simulink model "PassengerCar"  (R2019b)
settings: Solver=ode1  StartTime=0  StopTime=25  FixedStep=1.0000000000000000e-003  RelTol=1e-3
InitFcn:
  | sampleTime = str2double(get_param(bdroot, 'FixedStep'));
undefined symbols (not defined in the file or in its folder): AccPedalPos, BrakePedalPos, BrakeSwitch, DiscIntNeverNeededParam, DYNA4, EngSpd, IgnitionSwitch, InitialGear, InitialSpeed, IntendedEngTrq, LeftIndicator, MainBrakePress, MaxGear, MDL, MinGear, RefAcc, RefLane, RefLatPos, RefPath, RefPathCurv, RefSpd, RefSpdPreview, RefSpdRetrospect, RightIndicator, SteeringWheelAng, SteeringWheelTrq, UserDefinedRefValue, vm_const
libraries: UtilitiesLibrary x31, simulink x18, WheelSystemModules x13, LongitudinalControllerModules x13, LateralControllerModules x7, AnimationBusselectorModules x5, EnvironmentModules x5, BasicEngineControlModules x5, MiscellaneousControlModules x5, Animation3Modules x4, AuxiliariesModules x4, TireModules x4
(part 16 of 39)

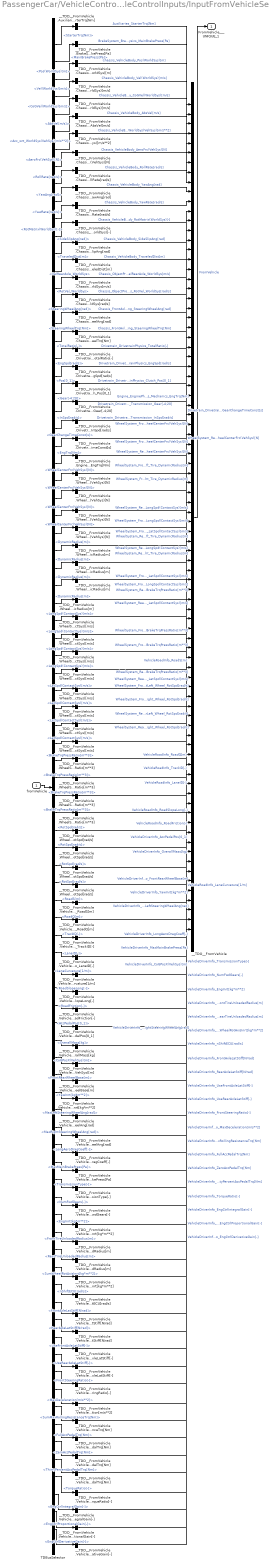
== system PassengerCar/VehicleControl/VehicleControlInputs/InputFromVehicleSelection ==
  fromVehicle : Inport
  TDBusSelector : BusSelector  OutputSignals=Auxiliaries.StarterTrq[Nm],BrakeSystem.BrakeSystemPhysics.MainBrakePress[Pa],Chassis.VehicleBody.Pos(WorldSys)[m],Chassis.VehicleBody.Vel(WorldSys)[m/s],Chassis.VehicleBody.CoGVel(WorldSys)[m/s],Chassis.VehicleBody.AbsVel[m/s],Chassis.VehicleBody.Acc_wrt_WorldSys(VehSys)[m/s**2],Chassis.VehicleBody.AeroFrc(VehSys)[N],Chassis.VehicleBody.RollRate[rad/s],Chassis.VehicleBody.YawAng[rad],Chassis.VehicleBody.YawRate[rad/s],Chassis.VehicleBody.RotMatrix(WorldSys)[-],Chassis.VehicleBody.SideSlipAng[rad],Chassis.VehicleBody.TraveledDist[m],Chassis.ObjectProperties.VelRearAxle_WorldSys,Chassis.ObjectProperties.RotVel_WorldSys,Chassis.FrontAxle.Steering.SteeringWheelAng[rad],Chassis.FrontAxle.Steering.SteeringWheelTrq[Nm],Drivetrain.DrivetrainPhysics.TotalRatio[-],Drivetrain.DrivetrainPhysics.EngSpd[rad/s],Drivetrain.DrivetrainPhysics.Clutch.Pos[0_1],Drivetrain.DrivetrainPhysics.Transmission.Gear[-4;20],Drivetrain.DrivetrainPhysics.Transmission.InSpd[rad/s],Drivetrain.DrivetrainPhysics.Transmission.GearChangeTimeConst[s],Engine.EnginePhysics.Mechanics.EngTrq[Nm],WheelSystem.FrontLeft.Tire.WheelCenterFrc(VehSys)[N],WheelSystem.FrontRight.Tire.WheelCenterFrc(VehSys)[N],WheelSystem.RearLeft.Tire.WheelCenterFrc(VehSys)[N],WheelSystem.RearRight.Tire.WheelCenterFrc(VehSys)[N],WheelSystem.FrontLeft.Tire.DynamicRadius[m],WheelSystem.FrontRight.Tire.DynamicRadius[m],WheelSystem.RearLeft.Tire.DynamicRadius[m],WheelSystem.RearRight.Tire.DynamicRadius[m],WheelSystem.FrontLeft.Tire.LongSpd(ContactSys)[m/s],WheelSystem.FrontRight.Tire.LongSpd(ContactSys)[m/s],WheelSystem.RearLeft.Tire.LongSpd(ContactSys)[m/s],WheelSystem.RearRight.Tire.LongSpd(ContactSys)[m/s],WheelSystem.FrontLeft.Tire.LatSpd(ContactSys)[m/s],WheelSystem.FrontRight.Tire.LatSpd(ContactSys)[m/s],WheelSystem.RearLeft.Tire.LatSpd(ContactSys)[m/s],WheelSystem.RearRight.Tire.LatSpd(ContactSys)[m/s],WheelSystem.FrontLeft.Wheel.BrakeTrqPressRatio[m**3],WheelSystem.FrontRight.Wheel.BrakeTrqPressRatio[m**3],WheelSystem.RearLeft.Wheel.BrakeTrqPressRatio[m**3],WheelSystem.RearRight.Wheel.BrakeTrqPressRatio[m**3],WheelSystem.FrontLeft.Wheel.RotSpd[rad/s],WheelSystem.FrontRight.Wheel.RotSpd[rad/s],WheelSystem.RearLeft.Wheel.RotSpd[rad/s],WheelSystem.RearRight.Wheel.RotSpd[rad/s],VehicleRoadInfo.RoadS[m],VehicleRoadInfo.RoadQ[m],VehicleRoadInfo.TrackID[-],VehicleRoadInfo.LaneID[-],VehicleRoadInfo.LaneCurvature[1/m],VehicleRoadInfo.RoadSlopeLong[-],VehicleRoadInfo.RoadFriction[-],VehicleDriverInfo.AccPedalPos[0_1],VehicleDriverInfo.OverallMass[kg],VehicleDriverInfo.CoGPosX(VehSys)[m],VehicleDriverInfo.FrontRearWheelBase[m],VehicleDriverInfo.YawInrt[kg*m**2],VehicleDriverInfo.MaxLeftSteeringWheelAng[rad],VehicleDriverInfo.MaxRightSteeringWheelAng[rad],VehicleDriverInfo.LongAeroDragCoeff[-],VehicleDriverInfo.MaxMainBrakePress[Pa],VehicleDriverInfo.TransmissionType[-],VehicleDriverInfo.NumFwdGears[-],VehicleDriverInfo.EngInrt[kg*m**2],VehicleDriverInfo.FrontTireUnloadedRadius[m],VehicleDriverInfo.RearTireUnloadedRadius[m],VehicleDriverInfo.SumWheelRotAxisInrt[kg*m**2],VehicleDriverInfo.nShiftECU[rad/s],VehicleDriverInfo.FrontAxleLatStiff[N/rad],VehicleDriverInfo.RearAxleLatStiff[N/rad],VehicleDriverInfo.UseFrontAxleLatStiff[-],VehicleDriverInfo.UseRearAxleLatStiff[-],VehicleDriverInfo.FrontSteeringRatio[-],VehicleDriverInfo.MaxDeceleration[m/s**2],VehicleDriverInfo.SumMaxRollingResistanceTrq[Nm],VehicleDriverInfo.FullAccPedalTrq[Nm],VehicleDriverInfo.ZeroAccPedalTrq[Nm],VehicleDriverInfo.ThirtyPercentAccPedalTrq[Nm],VehicleDriverInfo.TorqueRatio[-],VehicleDriverInfo.EngCtrlIntegralGain[-],VehicleDriverInfo.EngCtrlProportionalGain[-],VehicleDriverInfo.EngCtrlDerivativeGain[-]
  __TDD__FromVehicle.Auxiliaries_StarterTrq[Nm] : Demux  Outputs=[1]
  __TDD__FromVehicle.BrakeSystem_BrakeSystemPhysics_MainBrakePress[Pa] : Demux  Outputs=[1]
  __TDD__FromVehicle.Chassis_FrontAxle_Steering_SteeringWheelAng[rad] : Demux  Outputs=[1]
  __TDD__FromVehicle.Chassis_FrontAxle_Steering_SteeringWheelTrq[Nm] : Demux  Outputs=1
  __TDD__FromVehicle.Chassis_ObjectProperties_RotVel_WorldSys[rad/s] : Demux  Outputs=[3]
  __TDD__FromVehicle.Chassis_ObjectProperties_VelRearAxle_WorldSys[m/s] : Demux  Outputs=[3]
  __TDD__FromVehicle.Chassis_VehicleBody_AbsVel[m/s] : Demux  Outputs=[1]
  __TDD__FromVehicle.Chassis_VehicleBody_Acc_wrt_WorldSys(VehSys)[m/s**2] : Demux  Outputs=[3]
  __TDD__FromVehicle.Chassis_VehicleBody_AeroFrc(VehSys)[N] : Demux  Outputs=[3]
  __TDD__FromVehicle.Chassis_VehicleBody_CoGVel(WorldSys)[m/s] : Demux  Outputs=[3]
  __TDD__FromVehicle.Chassis_VehicleBody_Pos(WorldSys)[m] : Demux  Outputs=[3]
  __TDD__FromVehicle.Chassis_VehicleBody_RollRate[rad/s] : Demux  Outputs=[1]
  __TDD__FromVehicle.Chassis_VehicleBody_RotMatrix(WorldSys)[-] : Demux  Outputs=[9]
  __TDD__FromVehicle.Chassis_VehicleBody_SideSlipAng[rad] : Demux  Outputs=[1]
  __TDD__FromVehicle.Chassis_VehicleBody_TraveledDist[m] : Demux  Outputs=[1]
  __TDD__FromVehicle.Chassis_VehicleBody_Vel(WorldSys)[m/s] : Demux  Outputs=[3]
  __TDD__FromVehicle.Chassis_VehicleBody_YawAng[rad] : Demux  Outputs=[1]
  __TDD__FromVehicle.Chassis_VehicleBody_YawRate[rad/s] : Demux  Outputs=[1]
  __TDD__FromVehicle.Drivetrain_DrivetrainPhysics_Clutch_Pos[0_1] : Demux  Outputs=[1]
  __TDD__FromVehicle.Drivetrain_DrivetrainPhysics_EngSpd[rad/s] : Demux  Outputs=[1]
  __TDD__FromVehicle.Drivetrain_DrivetrainPhysics_TotalRatio[-] : Demux  Outputs=[1]
  __TDD__FromVehicle.Drivetrain_DrivetrainPhysics_Transmission_GearChangeTimeConst[s] : Demux  Outputs=[1]
  __TDD__FromVehicle.Drivetrain_DrivetrainPhysics_Transmission_Gear[-4;20] : Demux  Outputs=[1]
  __TDD__FromVehicle.Drivetrain_DrivetrainPhysics_Transmission_InSpd[rad/s] : Demux  Outputs=[1]
  __TDD__FromVehicle.Engine_EnginePhysics_Mechanics_EngTrq[Nm] : Demux  Outputs=[1]
  __TDD__FromVehicle.VehicleDriverInfo_AccPedalPos[0_1] : Demux  Outputs=[1]
  __TDD__FromVehicle.VehicleDriverInfo_CoGPosX(VehSys)[m] : Demux  Outputs=[1]
  __TDD__FromVehicle.VehicleDriverInfo_EngCtrlDerivativeGain[-] : Demux  Outputs=[1]
  __TDD__FromVehicle.VehicleDriverInfo_EngCtrlIntegralGain[-] : Demux  Outputs=[1]
  __TDD__FromVehicle.VehicleDriverInfo_EngCtrlProportionalGain[-] : Demux  Outputs=[1]
  __TDD__FromVehicle.VehicleDriverInfo_EngInrt[kg*m**2] : Demux  Outputs=[1]
  __TDD__FromVehicle.VehicleDriverInfo_FrontAxleLatStiff[N/rad] : Demux  Outputs=[1]
  __TDD__FromVehicle.VehicleDriverInfo_FrontRearWheelBase[m] : Demux  Outputs=[1]
  __TDD__FromVehicle.VehicleDriverInfo_FrontSteeringRatio[-] : Demux  Outputs=[1]
  __TDD__FromVehicle.VehicleDriverInfo_FrontTireUnloadedRadius[m] : Demux  Outputs=[1]
  __TDD__FromVehicle.VehicleDriverInfo_FullAccPedalTrq[Nm] : Demux  Outputs=[1]
  __TDD__FromVehicle.VehicleDriverInfo_LongAeroDragCoeff[-] : Demux  Outputs=[1]
  __TDD__FromVehicle.VehicleDriverInfo_MaxDeceleration[m/s**2] : Demux  Outputs=[1]
  __TDD__FromVehicle.VehicleDriverInfo_MaxLeftSteeringWheelAng[rad] : Demux  Outputs=[1]
  __TDD__FromVehicle.VehicleDriverInfo_MaxMainBrakePress[Pa] : Demux  Outputs=[1]
  __TDD__FromVehicle.VehicleDriverInfo_MaxRightSteeringWheelAng[rad] : Demux  Outputs=[1]
  __TDD__FromVehicle.VehicleDriverInfo_NumFwdGears[-] : Demux  Outputs=[1]
  __TDD__FromVehicle.VehicleDriverInfo_OverallMass[kg] : Demux  Outputs=[1]
  __TDD__FromVehicle.VehicleDriverInfo_RearAxleLatStiff[N/rad] : Demux  Outputs=[1]
  __TDD__FromVehicle.VehicleDriverInfo_RearTireUnloadedRadius[m] : Demux  Outputs=[1]
  __TDD__FromVehicle.VehicleDriverInfo_SumMaxRollingResistanceTrq[Nm] : Demux  Outputs=[1]
  __TDD__FromVehicle.VehicleDriverInfo_SumWheelRotAxisInrt[kg*m**2] : Demux  Outputs=[1]
  __TDD__FromVehicle.VehicleDriverInfo_ThirtyPercentAccPedalTrq[Nm] : Demux  Outputs=[1]
  __TDD__FromVehicle.VehicleDriverInfo_TorqueRatio[-] : Demux  Outputs=[1]
  __TDD__FromVehicle.VehicleDriverInfo_TransmissionType[-] : Demux  Outputs=[1]
  __TDD__FromVehicle.VehicleDriverInfo_UseFrontAxleLatStiff[-] : Demux  Outputs=[1]
  __TDD__FromVehicle.VehicleDriverInfo_UseRearAxleLatStiff[-] : Demux  Outputs=[1]
  __TDD__FromVehicle.VehicleDriverInfo_YawInrt[kg*m**2] : Demux  Outputs=[1]
  __TDD__FromVehicle.VehicleDriverInfo_ZeroAccPedalTrq[Nm] : Demux  Outputs=[1]
  __TDD__FromVehicle.VehicleDriverInfo_nShiftECU[rad/s] : Demux  Outputs=[1]
  __TDD__FromVehicle.VehicleRoadInfo_LaneCurvature[1/m] : Demux  Outputs=[1]
  __TDD__FromVehicle.VehicleRoadInfo_LaneID[-] : Demux  Outputs=[1]
  __TDD__FromVehicle.VehicleRoadInfo_RoadFriction[-] : Demux  Outputs=[1]
  __TDD__FromVehicle.VehicleRoadInfo_RoadQ[m] : Demux  Outputs=[1]
  __TDD__FromVehicle.VehicleRoadInfo_RoadS[m] : Demux  Outputs=[1]
  __TDD__FromVehicle.VehicleRoadInfo_RoadSlopeLong[-] : Demux  Outputs=[1]
  __TDD__FromVehicle.VehicleRoadInfo_TrackID[-] : Demux  Outputs=[1]
  __TDD__FromVehicle.WheelSystem_FrontLeft_Tire_DynamicRadius[m] : Demux  Outputs=[1]
  __TDD__FromVehicle.WheelSystem_FrontLeft_Tire_LatSpd(ContactSys)[m/s] : Demux  Outputs=[1]
  __TDD__FromVehicle.WheelSystem_FrontLeft_Tire_LongSpd(ContactSys)[m/s] : Demux  Outputs=[1]
  __TDD__FromVehicle.WheelSystem_FrontLeft_Tire_WheelCenterFrc(VehSys)[N] : Demux  Outputs=[3]
  __TDD__FromVehicle.WheelSystem_FrontLeft_Wheel_BrakeTrqPressRatio[m**3] : Demux  Outputs=[1]
  __TDD__FromVehicle.WheelSystem_FrontLeft_Wheel_RotSpd[rad/s] : Demux  Outputs=[1]
  __TDD__FromVehicle.WheelSystem_FrontRight_Tire_DynamicRadius[m] : Demux  Outputs=[1]
  __TDD__FromVehicle.WheelSystem_FrontRight_Tire_LatSpd(ContactSys)[m/s] : Demux  Outputs=[1]
  __TDD__FromVehicle.WheelSystem_FrontRight_Tire_LongSpd(ContactSys)[m/s] : Demux  Outputs=[1]
  __TDD__FromVehicle.WheelSystem_FrontRight_Tire_WheelCenterFrc(VehSys)[N] : Demux  Outputs=[3]
  __TDD__FromVehicle.WheelSystem_FrontRight_Wheel_BrakeTrqPressRatio[m**3] : Demux  Outputs=[1]
  __TDD__FromVehicle.WheelSystem_FrontRight_Wheel_RotSpd[rad/s] : Demux  Outputs=[1]
  __TDD__FromVehicle.WheelSystem_RearLeft_Tire_DynamicRadius[m] : Demux  Outputs=[1]
  __TDD__FromVehicle.WheelSystem_RearLeft_Tire_LatSpd(ContactSys)[m/s] : Demux  Outputs=[1]
  __TDD__FromVehicle.WheelSystem_RearLeft_Tire_LongSpd(ContactSys)[m/s] : Demux  Outputs=[1]
  __TDD__FromVehicle.WheelSystem_RearLeft_Tire_WheelCenterFrc(VehSys)[N] : Demux  Outputs=[3]
  __TDD__FromVehicle.WheelSystem_RearLeft_Wheel_BrakeTrqPressRatio[m**3] : Demux  Outputs=[1]
  __TDD__FromVehicle.WheelSystem_RearLeft_Wheel_RotSpd[rad/s] : Demux  Outputs=[1]
  __TDD__FromVehicle.WheelSystem_RearRight_Tire_DynamicRadius[m] : Demux  Outputs=[1]
  __TDD__FromVehicle.WheelSystem_RearRight_Tire_LatSpd(ContactSys)[m/s] : Demux  Outputs=[1]
  __TDD__FromVehicle.WheelSystem_RearRight_Tire_LongSpd(ContactSys)[m/s] : Demux  Outputs=[1]
  __TDD__FromVehicle.WheelSystem_RearRight_Tire_WheelCenterFrc(VehSys)[N] : Demux  Outputs=[3]
  __TDD__FromVehicle.WheelSystem_RearRight_Wheel_BrakeTrqPressRatio[m**3] : Demux  Outputs=[1]
  __TDD__FromVehicle.WheelSystem_RearRight_Wheel_RotSpd[rad/s] : Demux  Outputs=[1]
  __TDO__FromVehicle : BusCreator  Inputs=86
  FromVehicle___UNIQUE_1 : Outport  Description=|  VectorParamsAs1DForOutWhenUnconnected=off
      | <name>Auxiliaries.StarterTrq[Nm]</name>
      | <comment>Starter torque</comment>
  wires:
  __TDO__FromVehicle/1 -> FromVehicle___UNIQUE_1/1  "FromVehicle"
  __TDD__FromVehicle.VehicleDriverInfo_EngCtrlDerivativeGain[-]/1 -> __TDO__FromVehicle/86  "VehicleDriverInfo_EngCtrlDerivativeGain[-]"
  TDBusSelector/86 -> __TDD__FromVehicle.VehicleDriverInfo_EngCtrlDerivativeGain[-]/1  "<EngCtrlDerivativeGain[-]>"
  __TDD__FromVehicle.VehicleDriverInfo_EngCtrlProportionalGain[-]/1 -> __TDO__FromVehicle/85  "VehicleDriverInfo_EngCtrlProportionalGain[-]"
  TDBusSelector/85 -> __TDD__FromVehicle.VehicleDriverInfo_EngCtrlProportionalGain[-]/1  "<EngCtrlProportionalGain[-]>"
  __TDD__FromVehicle.VehicleDriverInfo_EngCtrlIntegralGain[-]/1 -> __TDO__FromVehicle/84  "VehicleDriverInfo_EngCtrlIntegralGain[-]"
  TDBusSelector/84 -> __TDD__FromVehicle.VehicleDriverInfo_EngCtrlIntegralGain[-]/1  "<EngCtrlIntegralGain[-]>"
  __TDD__FromVehicle.VehicleDriverInfo_TorqueRatio[-]/1 -> __TDO__FromVehicle/83  "VehicleDriverInfo_TorqueRatio[-]"
  TDBusSelector/83 -> __TDD__FromVehicle.VehicleDriverInfo_TorqueRatio[-]/1  "<TorqueRatio[-]>"
  __TDD__FromVehicle.VehicleDriverInfo_ThirtyPercentAccPedalTrq[Nm]/1 -> __TDO__FromVehicle/82  "VehicleDriverInfo_ThirtyPercentAccPedalTrq[Nm]"
  TDBusSelector/82 -> __TDD__FromVehicle.VehicleDriverInfo_ThirtyPercentAccPedalTrq[Nm]/1  "<ThirtyPercentAccPedalTrq[Nm]>"
  __TDD__FromVehicle.VehicleDriverInfo_ZeroAccPedalTrq[Nm]/1 -> __TDO__FromVehicle/81  "VehicleDriverInfo_ZeroAccPedalTrq[Nm]"
  TDBusSelector/81 -> __TDD__FromVehicle.VehicleDriverInfo_ZeroAccPedalTrq[Nm]/1  "<ZeroAccPedalTrq[Nm]>"
  __TDD__FromVehicle.VehicleDriverInfo_FullAccPedalTrq[Nm]/1 -> __TDO__FromVehicle/80  "VehicleDriverInfo_FullAccPedalTrq[Nm]"
  TDBusSelector/80 -> __TDD__FromVehicle.VehicleDriverInfo_FullAccPedalTrq[Nm]/1  "<FullAccPedalTrq[Nm]>"
  __TDD__FromVehicle.VehicleDriverInfo_SumMaxRollingResistanceTrq[Nm]/1 -> __TDO__FromVehicle/79  "VehicleDriverInfo_SumMaxRollingResistanceTrq[Nm]"
  TDBusSelector/79 -> __TDD__FromVehicle.VehicleDriverInfo_SumMaxRollingResistanceTrq[Nm]/1  "<SumMaxRollingResistanceTrq[Nm]>"
  __TDD__FromVehicle.VehicleDriverInfo_MaxDeceleration[m/s**2]/1 -> __TDO__FromVehicle/78  "VehicleDriverInfo_MaxDeceleration[m/s**2]"
  TDBusSelector/78 -> __TDD__FromVehicle.VehicleDriverInfo_MaxDeceleration[m/s**2]/1  "<MaxDeceleration[m/s**2]>"
  __TDD__FromVehicle.VehicleDriverInfo_FrontSteeringRatio[-]/1 -> __TDO__FromVehicle/77  "VehicleDriverInfo_FrontSteeringRatio[-]"
  TDBusSelector/77 -> __TDD__FromVehicle.VehicleDriverInfo_FrontSteeringRatio[-]/1  "<FrontSteeringRatio[-]>"
  __TDD__FromVehicle.VehicleDriverInfo_UseRearAxleLatStiff[-]/1 -> __TDO__FromVehicle/76  "VehicleDriverInfo_UseRearAxleLatStiff[-]"
  TDBusSelector/76 -> __TDD__FromVehicle.VehicleDriverInfo_UseRearAxleLatStiff[-]/1  "<UseRearAxleLatStiff[-]>"
  __TDD__FromVehicle.VehicleDriverInfo_UseFrontAxleLatStiff[-]/1 -> __TDO__FromVehicle/75  "VehicleDriverInfo_UseFrontAxleLatStiff[-]"
  TDBusSelector/75 -> __TDD__FromVehicle.VehicleDriverInfo_UseFrontAxleLatStiff[-]/1  "<UseFrontAxleLatStiff[-]>"
  __TDD__FromVehicle.VehicleDriverInfo_RearAxleLatStiff[N/rad]/1 -> __TDO__FromVehicle/74  "VehicleDriverInfo_RearAxleLatStiff[N/rad]"
  TDBusSelector/74 -> __TDD__FromVehicle.VehicleDriverInfo_RearAxleLatStiff[N/rad]/1  "<RearAxleLatStiff[N/rad]>"
  __TDD__FromVehicle.VehicleDriverInfo_FrontAxleLatStiff[N/rad]/1 -> __TDO__FromVehicle/73  "VehicleDriverInfo_FrontAxleLatStiff[N/rad]"
  TDBusSelector/73 -> __TDD__FromVehicle.VehicleDriverInfo_FrontAxleLatStiff[N/rad]/1  "<FrontAxleLatStiff[N/rad]>"
  __TDD__FromVehicle.VehicleDriverInfo_nShiftECU[rad/s]/1 -> __TDO__FromVehicle/72  "VehicleDriverInfo_nShiftECU[rad/s]"
  TDBusSelector/72 -> __TDD__FromVehicle.VehicleDriverInfo_nShiftECU[rad/s]/1  "<nShiftECU[rad/s]>"
  __TDD__FromVehicle.VehicleDriverInfo_SumWheelRotAxisInrt[kg*m**2]/1 -> __TDO__FromVehicle/71  "VehicleDriverInfo_SumWheelRotAxisInrt[kg*m**2]"
  TDBusSelector/71 -> __TDD__FromVehicle.VehicleDriverInfo_SumWheelRotAxisInrt[kg*m**2]/1  "<SumWheelRotAxisInrt[kg*m**2]>"
  __TDD__FromVehicle.VehicleDriverInfo_RearTireUnloadedRadius[m]/1 -> __TDO__FromVehicle/70  "VehicleDriverInfo_RearTireUnloadedRadius[m]"
  TDBusSelector/70 -> __TDD__FromVehicle.VehicleDriverInfo_RearTireUnloadedRadius[m]/1  "<RearTireUnloadedRadius[m]>"
  __TDD__FromVehicle.VehicleDriverInfo_FrontTireUnloadedRadius[m]/1 -> __TDO__FromVehicle/69  "VehicleDriverInfo_FrontTireUnloadedRadius[m]"
  TDBusSelector/69 -> __TDD__FromVehicle.VehicleDriverInfo_FrontTireUnloadedRadius[m]/1  "<FrontTireUnloadedRadius[m]>"
  __TDD__FromVehicle.VehicleDriverInfo_EngInrt[kg*m**2]/1 -> __TDO__FromVehicle/68  "VehicleDriverInfo_EngInrt[kg*m**2]"
  TDBusSelector/68 -> __TDD__FromVehicle.VehicleDriverInfo_EngInrt[kg*m**2]/1  "<EngInrt[kg*m**2]>"
  __TDD__FromVehicle.VehicleDriverInfo_NumFwdGears[-]/1 -> __TDO__FromVehicle/67  "VehicleDriverInfo_NumFwdGears[-]"
  TDBusSelector/67 -> __TDD__FromVehicle.VehicleDriverInfo_NumFwdGears[-]/1  "<NumFwdGears[-]>"
  __TDD__FromVehicle.VehicleDriverInfo_TransmissionType[-]/1 -> __TDO__FromVehicle/66  "VehicleDriverInfo_TransmissionType[-]"
  TDBusSelector/66 -> __TDD__FromVehicle.VehicleDriverInfo_TransmissionType[-]/1  "<TransmissionType[-]>"
  __TDD__FromVehicle.VehicleDriverInfo_MaxMainBrakePress[Pa]/1 -> __TDO__FromVehicle/65  "VehicleDriverInfo_MaxMainBrakePress[Pa]"
  TDBusSelector/65 -> __TDD__FromVehicle.VehicleDriverInfo_MaxMainBrakePress[Pa]/1  "<MaxMainBrakePress[Pa]>"
  __TDD__FromVehicle.VehicleDriverInfo_LongAeroDragCoeff[-]/1 -> __TDO__FromVehicle/64  "VehicleDriverInfo_LongAeroDragCoeff[-]"
  TDBusSelector/64 -> __TDD__FromVehicle.VehicleDriverInfo_LongAeroDragCoeff[-]/1  "<LongAeroDragCoeff[-]>"
  __TDD__FromVehicle.VehicleDriverInfo_MaxRightSteeringWheelAng[rad]/1 -> __TDO__FromVehicle/63  "VehicleDriverInfo_MaxRightSteeringWheelAng[rad]"
  TDBusSelector/63 -> __TDD__FromVehicle.VehicleDriverInfo_MaxRightSteeringWheelAng[rad]/1  "<MaxRightSteeringWheelAng[rad]>"
  __TDD__FromVehicle.VehicleDriverInfo_MaxLeftSteeringWheelAng[rad]/1 -> __TDO__FromVehicle/62  "VehicleDriverInfo_MaxLeftSteeringWheelAng[rad]"
  TDBusSelector/62 -> __TDD__FromVehicle.VehicleDriverInfo_MaxLeftSteeringWheelAng[rad]/1  "<MaxLeftSteeringWheelAng[rad]>"
  __TDD__FromVehicle.VehicleDriverInfo_YawInrt[kg*m**2]/1 -> __TDO__FromVehicle/61  "VehicleDriverInfo_YawInrt[kg*m**2]"
  TDBusSelector/61 -> __TDD__FromVehicle.VehicleDriverInfo_YawInrt[kg*m**2]/1  "<YawInrt[kg*m**2]>"
  __TDD__FromVehicle.VehicleDriverInfo_FrontRearWheelBase[m]/1 -> __TDO__FromVehicle/60  "VehicleDriverInfo_FrontRearWheelBase[m]"
  TDBusSelector/60 -> __TDD__FromVehicle.VehicleDriverInfo_FrontRearWheelBase[m]/1  "<FrontRearWheelBase[m]>"
  __TDD__FromVehicle.VehicleDriverInfo_CoGPosX(VehSys)[m]/1 -> __TDO__FromVehicle/59  "VehicleDriverInfo_CoGPosX(VehSys)[m]"
  TDBusSelector/59 -> __TDD__FromVehicle.VehicleDriverInfo_CoGPosX(VehSys)[m]/1  "<CoGPosX(VehSys)[m]>"
  __TDD__FromVehicle.VehicleDriverInfo_OverallMass[kg]/1 -> __TDO__FromVehicle/58  "VehicleDriverInfo_OverallMass[kg]"
  TDBusSelector/58 -> __TDD__FromVehicle.VehicleDriverInfo_OverallMass[kg]/1  "<OverallMass[kg]>"
  __TDD__FromVehicle.VehicleDriverInfo_AccPedalPos[0_1]/1 -> __TDO__FromVehicle/57  "VehicleDriverInfo_AccPedalPos[0_1]"
  TDBusSelector/57 -> __TDD__FromVehicle.VehicleDriverInfo_AccPedalPos[0_1]/1  "<AccPedalPos[0_1]>"
  __TDD__FromVehicle.VehicleRoadInfo_RoadFriction[-]/1 -> __TDO__FromVehicle/56  "VehicleRoadInfo_RoadFriction[-]"
  TDBusSelector/56 -> __TDD__FromVehicle.VehicleRoadInfo_RoadFriction[-]/1  "<RoadFriction[-]>"
  __TDD__FromVehicle.VehicleRoadInfo_RoadSlopeLong[-]/1 -> __TDO__FromVehicle/55  "VehicleRoadInfo_RoadSlopeLong[-]"
  TDBusSelector/55 -> __TDD__FromVehicle.VehicleRoadInfo_RoadSlopeLong[-]/1  "<RoadSlopeLong[-]>"
  __TDD__FromVehicle.VehicleRoadInfo_LaneCurvature[1/m]/1 -> __TDO__FromVehicle/54  "VehicleRoadInfo_LaneCurvature[1/m]"
  TDBusSelector/54 -> __TDD__FromVehicle.VehicleRoadInfo_LaneCurvature[1/m]/1  "<LaneCurvature[1/m]>"
  __TDD__FromVehicle.VehicleRoadInfo_LaneID[-]/1 -> __TDO__FromVehicle/53  "VehicleRoadInfo_LaneID[-]"
  TDBusSelector/53 -> __TDD__FromVehicle.VehicleRoadInfo_LaneID[-]/1  "<LaneID[-]>"
  __TDD__FromVehicle.VehicleRoadInfo_TrackID[-]/1 -> __TDO__FromVehicle/52  "VehicleRoadInfo_TrackID[-]"
  TDBusSelector/52 -> __TDD__FromVehicle.VehicleRoadInfo_TrackID[-]/1  "<TrackID[-]>"
  __TDD__FromVehicle.VehicleRoadInfo_RoadQ[m]/1 -> __TDO__FromVehicle/51  "VehicleRoadInfo_RoadQ[m]"
  TDBusSelector/51 -> __TDD__FromVehicle.VehicleRoadInfo_RoadQ[m]/1  "<RoadQ[m]>"
  __TDD__FromVehicle.VehicleRoadInfo_RoadS[m]/1 -> __TDO__FromVehicle/50  "VehicleRoadInfo_RoadS[m]"
  TDBusSelector/50 -> __TDD__FromVehicle.VehicleRoadInfo_RoadS[m]/1  "<RoadS[m]>"
  __TDD__FromVehicle.WheelSystem_RearRight_Wheel_RotSpd[rad/s]/1 -> __TDO__FromVehicle/49  "WheelSystem_RearRight_Wheel_RotSpd[rad/s]"
  TDBusSelector/49 -> __TDD__FromVehicle.WheelSystem_RearRight_Wheel_RotSpd[rad/s]/1  "<RotSpd[rad/s]>"
  __TDD__FromVehicle.WheelSystem_RearLeft_Wheel_RotSpd[rad/s]/1 -> __TDO__FromVehicle/48  "WheelSystem_RearLeft_Wheel_RotSpd[rad/s]"
  TDBusSelector/48 -> __TDD__FromVehicle.WheelSystem_RearLeft_Wheel_RotSpd[rad/s]/1  "<RotSpd[rad/s]>"
  __TDD__FromVehicle.WheelSystem_FrontRight_Wheel_RotSpd[rad/s]/1 -> __TDO__FromVehicle/47  "WheelSystem_FrontRight_Wheel_RotSpd[rad/s]"
  TDBusSelector/47 -> __TDD__FromVehicle.WheelSystem_FrontRight_Wheel_RotSpd[rad/s]/1  "<RotSpd[rad/s]>"
  __TDD__FromVehicle.WheelSystem_FrontLeft_Wheel_RotSpd[rad/s]/1 -> __TDO__FromVehicle/46  "WheelSystem_FrontLeft_Wheel_RotSpd[rad/s]"
  TDBusSelector/46 -> __TDD__FromVehicle.WheelSystem_FrontLeft_Wheel_RotSpd[rad/s]/1  "<RotSpd[rad/s]>"
  __TDD__FromVehicle.WheelSystem_RearRight_Wheel_BrakeTrqPressRatio[m**3]/1 -> __TDO__FromVehicle/45  "WheelSystem_RearRight_Wheel_BrakeTrqPressRatio[m**3]"
  TDBusSelector/45 -> __TDD__FromVehicle.WheelSystem_RearRight_Wheel_BrakeTrqPressRatio[m**3]/1  "<BrakeTrqPressRatio[m**3]>"
  __TDD__FromVehicle.WheelSystem_RearLeft_Wheel_BrakeTrqPressRatio[m**3]/1 -> __TDO__FromVehicle/44  "WheelSystem_RearLeft_Wheel_BrakeTrqPressRatio[m**3]"
  TDBusSelector/44 -> __TDD__FromVehicle.WheelSystem_RearLeft_Wheel_BrakeTrqPressRatio[m**3]/1  "<BrakeTrqPressRatio[m**3]>"
  __TDD__FromVehicle.WheelSystem_FrontRight_Wheel_BrakeTrqPressRatio[m**3]/1 -> __TDO__FromVehicle/43  "WheelSystem_FrontRight_Wheel_BrakeTrqPressRatio[m**3]"
  TDBusSelector/43 -> __TDD__FromVehicle.WheelSystem_FrontRight_Wheel_BrakeTrqPressRatio[m**3]/1  "<BrakeTrqPressRatio[m**3]>"
  __TDD__FromVehicle.WheelSystem_FrontLeft_Wheel_BrakeTrqPressRatio[m**3]/1 -> __TDO__FromVehicle/42  "WheelSystem_FrontLeft_Wheel_BrakeTrqPressRatio[m**3]"
  TDBusSelector/42 -> __TDD__FromVehicle.WheelSystem_FrontLeft_Wheel_BrakeTrqPressRatio[m**3]/1  "<BrakeTrqPressRatio[m**3]>"
  __TDD__FromVehicle.WheelSystem_RearRight_Tire_LatSpd(ContactSys)[m/s]/1 -> __TDO__FromVehicle/41  "WheelSystem_RearRight_Tire_LatSpd(ContactSys)[m/s]"
  TDBusSelector/41 -> __TDD__FromVehicle.WheelSystem_RearRight_Tire_LatSpd(ContactSys)[m/s]/1  "<LatSpd(ContactSys)[m/s]>"
  __TDD__FromVehicle.WheelSystem_RearLeft_Tire_LatSpd(ContactSys)[m/s]/1 -> __TDO__FromVehicle/40  "WheelSystem_RearLeft_Tire_LatSpd(ContactSys)[m/s]"
  TDBusSelector/40 -> __TDD__FromVehicle.WheelSystem_RearLeft_Tire_LatSpd(ContactSys)[m/s]/1  "<LatSpd(ContactSys)[m/s]>"
  __TDD__FromVehicle.WheelSystem_FrontRight_Tire_LatSpd(ContactSys)[m/s]/1 -> __TDO__FromVehicle/39  "WheelSystem_FrontRight_Tire_LatSpd(ContactSys)[m/s]"
  TDBusSelector/39 -> __TDD__FromVehicle.WheelSystem_FrontRight_Tire_LatSpd(ContactSys)[m/s]/1  "<LatSpd(ContactSys)[m/s]>"
  __TDD__FromVehicle.WheelSystem_FrontLeft_Tire_LatSpd(ContactSys)[m/s]/1 -> __TDO__FromVehicle/38  "WheelSystem_FrontLeft_Tire_LatSpd(ContactSys)[m/s]"
  TDBusSelector/38 -> __TDD__FromVehicle.WheelSystem_FrontLeft_Tire_LatSpd(ContactSys)[m/s]/1  "<LatSpd(ContactSys)[m/s]>"
  __TDD__FromVehicle.WheelSystem_RearRight_Tire_LongSpd(ContactSys)[m/s]/1 -> __TDO__FromVehicle/37  "WheelSystem_RearRight_Tire_LongSpd(ContactSys)[m/s]"
  TDBusSelector/37 -> __TDD__FromVehicle.WheelSystem_RearRight_Tire_LongSpd(ContactSys)[m/s]/1  "<LongSpd(ContactSys)[m/s]>"
  __TDD__FromVehicle.WheelSystem_RearLeft_Tire_LongSpd(ContactSys)[m/s]/1 -> __TDO__FromVehicle/36  "WheelSystem_RearLeft_Tire_LongSpd(ContactSys)[m/s]"
  TDBusSelector/36 -> __TDD__FromVehicle.WheelSystem_RearLeft_Tire_LongSpd(ContactSys)[m/s]/1  "<LongSpd(ContactSys)[m/s]>"
  __TDD__FromVehicle.WheelSystem_FrontRight_Tire_LongSpd(ContactSys)[m/s]/1 -> __TDO__FromVehicle/35  "WheelSystem_FrontRight_Tire_LongSpd(ContactSys)[m/s]"
  TDBusSelector/35 -> __TDD__FromVehicle.WheelSystem_FrontRight_Tire_LongSpd(ContactSys)[m/s]/1  "<LongSpd(ContactSys)[m/s]>"
  __TDD__FromVehicle.WheelSystem_FrontLeft_Tire_LongSpd(ContactSys)[m/s]/1 -> __TDO__FromVehicle/34  "WheelSystem_FrontLeft_Tire_LongSpd(ContactSys)[m/s]"
  TDBusSelector/34 -> __TDD__FromVehicle.WheelSystem_FrontLeft_Tire_LongSpd(ContactSys)[m/s]/1  "<LongSpd(ContactSys)[m/s]>"
  __TDD__FromVehicle.WheelSystem_RearRight_Tire_DynamicRadius[m]/1 -> __TDO__FromVehicle/33  "WheelSystem_RearRight_Tire_DynamicRadius[m]"
  TDBusSelector/33 -> __TDD__FromVehicle.WheelSystem_RearRight_Tire_DynamicRadius[m]/1  "<DynamicRadius[m]>"
  __TDD__FromVehicle.WheelSystem_RearLeft_Tire_DynamicRadius[m]/1 -> __TDO__FromVehicle/32  "WheelSystem_RearLeft_Tire_DynamicRadius[m]"
  TDBusSelector/32 -> __TDD__FromVehicle.WheelSystem_RearLeft_Tire_DynamicRadius[m]/1  "<DynamicRadius[m]>"
  __TDD__FromVehicle.WheelSystem_FrontRight_Tire_DynamicRadius[m]/1 -> __TDO__FromVehicle/31  "WheelSystem_FrontRight_Tire_DynamicRadius[m]"
  TDBusSelector/31 -> __TDD__FromVehicle.WheelSystem_FrontRight_Tire_DynamicRadius[m]/1  "<DynamicRadius[m]>"
  __TDD__FromVehicle.WheelSystem_FrontLeft_Tire_DynamicRadius[m]/1 -> __TDO__FromVehicle/30  "WheelSystem_FrontLeft_Tire_DynamicRadius[m]"
  TDBusSelector/30 -> __TDD__FromVehicle.WheelSystem_FrontLeft_Tire_DynamicRadius[m]/1  "<DynamicRadius[m]>"
  __TDD__FromVehicle.WheelSystem_RearRight_Tire_WheelCenterFrc(VehSys)[N]/1 -> __TDO__FromVehicle/29  "WheelSystem_RearRight_Tire_WheelCenterFrc(VehSys)[N]"
  TDBusSelector/29 -> __TDD__FromVehicle.WheelSystem_RearRight_Tire_WheelCenterFrc(VehSys)[N]/1  "<WheelCenterFrc(VehSys)[N]>"
  __TDD__FromVehicle.WheelSystem_RearLeft_Tire_WheelCenterFrc(VehSys)[N]/1 -> __TDO__FromVehicle/28  "WheelSystem_RearLeft_Tire_WheelCenterFrc(VehSys)[N]"
  TDBusSelector/28 -> __TDD__FromVehicle.WheelSystem_RearLeft_Tire_WheelCenterFrc(VehSys)[N]/1  "<WheelCenterFrc(VehSys)[N]>"
  __TDD__FromVehicle.WheelSystem_FrontRight_Tire_WheelCenterFrc(VehSys)[N]/1 -> __TDO__FromVehicle/27  "WheelSystem_FrontRight_Tire_WheelCenterFrc(VehSys)[N]"
  TDBusSelector/27 -> __TDD__FromVehicle.WheelSystem_FrontRight_Tire_WheelCenterFrc(VehSys)[N]/1  "<WheelCenterFrc(VehSys)[N]>"
  __TDD__FromVehicle.WheelSystem_FrontLeft_Tire_WheelCenterFrc(VehSys)[N]/1 -> __TDO__FromVehicle/26  "WheelSystem_FrontLeft_Tire_WheelCenterFrc(VehSys)[N]"
  TDBusSelector/26 -> __TDD__FromVehicle.WheelSystem_FrontLeft_Tire_WheelCenterFrc(VehSys)[N]/1  "<WheelCenterFrc(VehSys)[N]>"
  __TDD__FromVehicle.Engine_EnginePhysics_Mechanics_EngTrq[Nm]/1 -> __TDO__FromVehicle/25  "Engine_EnginePhysics_Mechanics_EngTrq[Nm]"
  TDBusSelector/25 -> __TDD__FromVehicle.Engine_EnginePhysics_Mechanics_EngTrq[Nm]/1  "<EngTrq[Nm]>"
  __TDD__FromVehicle.Drivetrain_DrivetrainPhysics_Transmission_GearChangeTimeConst[s]/1 -> __TDO__FromVehicle/24  "Drivetrain_DrivetrainPhysics_Transmission_GearChangeTimeConst[s]"
  TDBusSelector/24 -> __TDD__FromVehicle.Drivetrain_DrivetrainPhysics_Transmission_GearChangeTimeConst[s]/1  "<GearChangeTimeConst[s]>"
  __TDD__FromVehicle.Drivetrain_DrivetrainPhysics_Transmission_InSpd[rad/s]/1 -> __TDO__FromVehicle/23  "Drivetrain_DrivetrainPhysics_Transmission_InSpd[rad/s]"
  TDBusSelector/23 -> __TDD__FromVehicle.Drivetrain_DrivetrainPhysics_Transmission_InSpd[rad/s]/1  "<InSpd[rad/s]>"
  __TDD__FromVehicle.Drivetrain_DrivetrainPhysics_Transmission_Gear[-4;20]/1 -> __TDO__FromVehicle/22  "Drivetrain_DrivetrainPhysics_Transmission_Gear[-4;20]"
  TDBusSelector/22 -> __TDD__FromVehicle.Drivetrain_DrivetrainPhysics_Transmission_Gear[-4;20]/1  "<Gear[-4;20]>"
  __TDD__FromVehicle.Drivetrain_DrivetrainPhysics_Clutch_Pos[0_1]/1 -> __TDO__FromVehicle/21  "Drivetrain_DrivetrainPhysics_Clutch_Pos[0_1]"
  TDBusSelector/21 -> __TDD__FromVehicle.Drivetrain_DrivetrainPhysics_Clutch_Pos[0_1]/1  "<Pos[0_1]>"
  __TDD__FromVehicle.Drivetrain_DrivetrainPhysics_EngSpd[rad/s]/1 -> __TDO__FromVehicle/20  "Drivetrain_DrivetrainPhysics_EngSpd[rad/s]"
  TDBusSelector/20 -> __TDD__FromVehicle.Drivetrain_DrivetrainPhysics_EngSpd[rad/s]/1  "<EngSpd[rad/s]>"
  __TDD__FromVehicle.Drivetrain_DrivetrainPhysics_TotalRatio[-]/1 -> __TDO__FromVehicle/19  "Drivetrain_DrivetrainPhysics_TotalRatio[-]"
  TDBusSelector/19 -> __TDD__FromVehicle.Drivetrain_DrivetrainPhysics_TotalRatio[-]/1  "<TotalRatio[-]>"
  __TDD__FromVehicle.Chassis_FrontAxle_Steering_SteeringWheelTrq[Nm]/1 -> __TDO__FromVehicle/18  "Chassis_FrontAxle_Steering_SteeringWheelTrq[Nm]"
  TDBusSelector/18 -> __TDD__FromVehicle.Chassis_FrontAxle_Steering_SteeringWheelTrq[Nm]/1  "<SteeringWheelTrq[Nm]>"
  __TDD__FromVehicle.Chassis_FrontAxle_Steering_SteeringWheelAng[rad]/1 -> __TDO__FromVehicle/17  "Chassis_FrontAxle_Steering_SteeringWheelAng[rad]"
  TDBusSelector/17 -> __TDD__FromVehicle.Chassis_FrontAxle_Steering_SteeringWheelAng[rad]/1  "<SteeringWheelAng[rad]>"
  __TDD__FromVehicle.Chassis_ObjectProperties_RotVel_WorldSys[rad/s]/1 -> __TDO__FromVehicle/16  "Chassis_ObjectProperties_RotVel_WorldSys[rad/s]"
  TDBusSelector/16 -> __TDD__FromVehicle.Chassis_ObjectProperties_RotVel_WorldSys[rad/s]/1  "<RotVel_WorldSys>"
  __TDD__FromVehicle.Chassis_ObjectProperties_VelRearAxle_WorldSys[m/s]/1 -> __TDO__FromVehicle/15  "Chassis_ObjectProperties_VelRearAxle_WorldSys[m/s]"
  TDBusSelector/15 -> __TDD__FromVehicle.Chassis_ObjectProperties_VelRearAxle_WorldSys[m/s]/1  "<VelRearAxle_WorldSys>"
  __TDD__FromVehicle.Chassis_VehicleBody_TraveledDist[m]/1 -> __TDO__FromVehicle/14  "Chassis_VehicleBody_TraveledDist[m]"
  TDBusSelector/14 -> __TDD__FromVehicle.Chassis_VehicleBody_TraveledDist[m]/1  "<TraveledDist[m]>"
  __TDD__FromVehicle.Chassis_VehicleBody_SideSlipAng[rad]/1 -> __TDO__FromVehicle/13  "Chassis_VehicleBody_SideSlipAng[rad]"
  TDBusSelector/13 -> __TDD__FromVehicle.Chassis_VehicleBody_SideSlipAng[rad]/1  "<SideSlipAng[rad]>"
  __TDD__FromVehicle.Chassis_VehicleBody_RotMatrix(WorldSys)[-]/1 -> __TDO__FromVehicle/12  "Chassis_VehicleBody_RotMatrix(WorldSys)[-]"
  TDBusSelector/12 -> __TDD__FromVehicle.Chassis_VehicleBody_RotMatrix(WorldSys)[-]/1  "<RotMatrix(WorldSys)[-]>"
  __TDD__FromVehicle.Chassis_VehicleBody_YawRate[rad/s]/1 -> __TDO__FromVehicle/11  "Chassis_VehicleBody_YawRate[rad/s]"
  TDBusSelector/11 -> __TDD__FromVehicle.Chassis_VehicleBody_YawRate[rad/s]/1  "<YawRate[rad/s]>"
  __TDD__FromVehicle.Chassis_VehicleBody_YawAng[rad]/1 -> __TDO__FromVehicle/10  "Chassis_VehicleBody_YawAng[rad]"
  TDBusSelector/10 -> __TDD__FromVehicle.Chassis_VehicleBody_YawAng[rad]/1  "<YawAng[rad]>"
  __TDD__FromVehicle.Chassis_VehicleBody_RollRate[rad/s]/1 -> __TDO__FromVehicle/9  "Chassis_VehicleBody_RollRate[rad/s]"
  TDBusSelector/9 -> __TDD__FromVehicle.Chassis_VehicleBody_RollRate[rad/s]/1  "<RollRate[rad/s]>"
  __TDD__FromVehicle.Chassis_VehicleBody_AeroFrc(VehSys)[N]/1 -> __TDO__FromVehicle/8  "Chassis_VehicleBody_AeroFrc(VehSys)[N]"
  TDBusSelector/8 -> __TDD__FromVehicle.Chassis_VehicleBody_AeroFrc(VehSys)[N]/1  "<AeroFrc(VehSys)[N]>"
  __TDD__FromVehicle.Chassis_VehicleBody_Acc_wrt_WorldSys(VehSys)[m/s**2]/1 -> __TDO__FromVehicle/7  "Chassis_VehicleBody_Acc_wrt_WorldSys(VehSys)[m/s**2]"
  TDBusSelector/7 -> __TDD__FromVehicle.Chassis_VehicleBody_Acc_wrt_WorldSys(VehSys)[m/s**2]/1  "<Acc_wrt_WorldSys(VehSys)[m/s**2]>"
  __TDD__FromVehicle.Chassis_VehicleBody_AbsVel[m/s]/1 -> __TDO__FromVehicle/6  "Chassis_VehicleBody_AbsVel[m/s]"
  TDBusSelector/6 -> __TDD__FromVehicle.Chassis_VehicleBody_AbsVel[m/s]/1  "<AbsVel[m/s]>"
  __TDD__FromVehicle.Chassis_VehicleBody_CoGVel(WorldSys)[m/s]/1 -> __TDO__FromVehicle/5  "Chassis_VehicleBody_CoGVel(WorldSys)[m/s]"
  TDBusSelector/5 -> __TDD__FromVehicle.Chassis_VehicleBody_CoGVel(WorldSys)[m/s]/1  "<CoGVel(WorldSys)[m/s]>"
  __TDD__FromVehicle.Chassis_VehicleBody_Vel(WorldSys)[m/s]/1 -> __TDO__FromVehicle/4  "Chassis_VehicleBody_Vel(WorldSys)[m/s]"
  TDBusSelector/4 -> __TDD__FromVehicle.Chassis_VehicleBody_Vel(WorldSys)[m/s]/1  "<Vel(WorldSys)[m/s]>"
  __TDD__FromVehicle.Chassis_VehicleBody_Pos(WorldSys)[m]/1 -> __TDO__FromVehicle/3  "Chassis_VehicleBody_Pos(WorldSys)[m]"
  TDBusSelector/3 -> __TDD__FromVehicle.Chassis_VehicleBody_Pos(WorldSys)[m]/1  "<Pos(WorldSys)[m]>"
  __TDD__FromVehicle.BrakeSystem_BrakeSystemPhysics_MainBrakePress[Pa]/1 -> __TDO__FromVehicle/2  "BrakeSystem_BrakeSystemPhysics_MainBrakePress[Pa]"
  TDBusSelector/2 -> __TDD__FromVehicle.BrakeSystem_BrakeSystemPhysics_MainBrakePress[Pa]/1  "<MainBrakePress[Pa]>"
  __TDD__FromVehicle.Auxiliaries_StarterTrq[Nm]/1 -> __TDO__FromVehicle/1  "Auxiliaries_StarterTrq[Nm]"
  TDBusSelector/1 -> __TDD__FromVehicle.Auxiliaries_StarterTrq[Nm]/1  "<StarterTrq[Nm]>"
  fromVehicle/1 -> TDBusSelector/1

== system PassengerCar/Vehicle/BrakeSystem/BrakeSystemControlUnit/BasicElectronicStabilityControl ==
  MaxMainBrakePress[Pa] : Inport
  WheelBrakePressuresFromBrakeHydraulics[Pa]1 : Inport  Port=2
  ABSSwitchFromVehicleControl[0;1] : Inport  Port=3
  ESCSwitchFromVehicleControl[0;1] : Inport  Port=4
  FrontLeftWheelLongSpd(ContactSys)[m/s] : Inport  Port=5
  FrontLeftWheelRotSpd[rad/s] : Inport  Port=6
  FrontLeftWheelRotAcc[rad/s**2] : Inport  Port=7
  FrontLeftTireDynamicRadius[m] : Inport  Port=8
  FrontRightWheelLongSpd(ContactSys)[m/s] : Inport  Port=9
  FrontRightWheelRotSpd[rad/s] : Inport  Port=10
  FrontRightWheelRotAcc[rad/s**2] : Inport  Port=11
  FrontRightTireDynamicRadius[m] : Inport  Port=12
  RearLeftWheelLongSpd(ContactSys)[m/s] : Inport  Port=13
  RearLeftWheelRotSpd[rad/s] : Inport  Port=14
  RearLeftWheelRotAcc[rad/s**2] : Inport  Port=15
  RearLeftTireDynamicRadius[m] : Inport  Port=16
  RearRightWheelLongSpd(ContactSys)[m/s] : Inport  Port=17
  RearRightWheelRotSpd[rad/s] : Inport  Port=18
  RearRightWheelRotAcc[rad/s**2] : Inport  Port=19
  RearRightTireDynamicRadius[m] : Inport  Port=20
  FrontLeftTireRadius[m] : Inport  Port=21
  RearLeftTireRadius[m] : Inport  Port=22
  FrontBrakeTrqPressRatio[m**3] : Inport  Port=23
  RearBrakeTrqPressRatio[m**3] : Inport  Port=24
  Vel_wrt_WorldSys(VehSys)[m/s] : Inport  Port=25
  Acc_wrt_WorldSys(VehSys)[m/**s2] : Inport  Port=26
  YawRate[rad/s] : Inport  Port=27
  YawInertia[kgm2] : Inport  Port=28
  FrontWheelTrack[m] : Inport  Port=29
  RearWheelTrack[m] : Inport  Port=30
  BasicAntiLockBrakeControl : Subsystem
  BasicYawStabilityControl : Subsystem
  Switch : Switch  Criteria=u2 > Threshold  Threshold=0.5
  Switch1 : Switch  Criteria=u2 > Threshold  Threshold=0.5
  Vel_wrt_WorldSys(VehSys)[m/s]1 : InportShadow  Port=25
  WheelBrakePressuresFromBrakeHydraulics[Pa] : InportShadow  Port=2
  WheelBrakePressures[Pa] : Outport  VectorParamsAs1DForOutWhenUnconnected=off
  YawStabilityControlInfo : Outport  Port=2  VectorParamsAs1DForOutWhenUnconnected=off
  AntiLockBrakeSystemInfo : Outport  Port=3  VectorParamsAs1DForOutWhenUnconnected=off
  wires:
  BasicAntiLockBrakeControl/3(AntiLockBrakeSystemInfo) -> AntiLockBrakeSystemInfo/1
  Vel_wrt_WorldSys(VehSys)[m/s]1/1 -> BasicAntiLockBrakeControl/3(Vel_wrt_WorldSys(VehSys)[m/s])
  ABSSwitchFromVehicleControl[0;1]/1 -> BasicAntiLockBrakeControl/1(ABSSwitchFromVehicleControl[0;1])
  ESCSwitchFromVehicleControl[0;1]/1 -> BasicYawStabilityControl/1(ESCSwitch[0;1])
  MaxMainBrakePress[Pa]/1 -> BasicAntiLockBrakeControl/20(MaxMainBrakePress[Pa])
  RearRightTireDynamicRadius[m]/1 -> BasicAntiLockBrakeControl/19(RearRightTireDynamicRadius[m])
  RearRightWheelRotAcc[rad/s**2]/1 -> BasicAntiLockBrakeControl/18(RearRightWheelRotAcc[rad/s**2])
  RearRightWheelRotSpd[rad/s]/1 -> BasicAntiLockBrakeControl/17(RearRightWheelRotSpd[rad/s])
  RearRightWheelLongSpd(ContactSys)[m/s]/1 -> BasicAntiLockBrakeControl/16(RearRightWheelLongSpd(ContactSys)[m/s])
  RearLeftTireDynamicRadius[m]/1 -> BasicAntiLockBrakeControl/15(RearLeftTireDynamicRadius[m])
  RearLeftWheelRotAcc[rad/s**2]/1 -> BasicAntiLockBrakeControl/14(RearLeftWheelRotAcc[rad/s**2])
  RearLeftWheelRotSpd[rad/s]/1 -> BasicAntiLockBrakeControl/13(RearLeftWheelRotSpd[rad/s])
  RearLeftWheelLongSpd(ContactSys)[m/s]/1 -> BasicAntiLockBrakeControl/12(RearLeftWheelLongSpd(ContactSys)[m/s])
  FrontRightTireDynamicRadius[m]/1 -> BasicAntiLockBrakeControl/11(FrontRightTireDynamicRadius[m])
  FrontRightWheelRotAcc[rad/s**2]/1 -> BasicAntiLockBrakeControl/10(FrontRightWheelRotAcc[rad/s**2])
  FrontRightWheelRotSpd[rad/s]/1 -> BasicAntiLockBrakeControl/9(FrontRightWheelRotSpd[rad/s])
  FrontRightWheelLongSpd(ContactSys)[m/s]/1 -> BasicAntiLockBrakeControl/8(FrontRightWheelLongSpd(ContactSys)[m/s])
  FrontLeftTireDynamicRadius[m]/1 -> BasicAntiLockBrakeControl/7(FrontLeftTireDynamicRadius[m])
  FrontLeftWheelRotAcc[rad/s**2]/1 -> BasicAntiLockBrakeControl/6(FrontLeftWheelRotAcc[rad/s**2])
  FrontLeftWheelRotSpd[rad/s]/1 -> BasicAntiLockBrakeControl/5(FrontLeftWheelRotSpd[rad/s])
  FrontLeftWheelLongSpd(ContactSys)[m/s]/1 -> BasicAntiLockBrakeControl/4(FrontLeftWheelLongSpd(ContactSys)[m/s])
  RearBrakeTrqPressRatio[m**3]/1 -> BasicYawStabilityControl/12(RearBrakeTrqPressRatio[m**3])
  FrontBrakeTrqPressRatio[m**3]/1 -> BasicYawStabilityControl/11(FrontBrakeTrqPressRatio[m**3])
  RearLeftTireRadius[m]/1 -> BasicYawStabilityControl/10(RearLeftTireRadius[m])
  FrontLeftTireRadius[m]/1 -> BasicYawStabilityControl/9(FrontLeftTireRadius[m])
  RearWheelTrack[m]/1 -> BasicYawStabilityControl/8(RearWheelTrack[m])
  FrontWheelTrack[m]/1 -> BasicYawStabilityControl/7(FrontWheelTrack[m])
  YawInertia[kgm2]/1 -> BasicYawStabilityControl/6(YawInertia[kgm2])
  YawRate[rad/s]/1 -> BasicYawStabilityControl/5(YawRate[rad/s])
  Acc_wrt_WorldSys(VehSys)[m/**s2]/1 -> BasicYawStabilityControl/4(Acc_wrt_WorldSys(VehSys)[m/**s2])
  Vel_wrt_WorldSys(VehSys)[m/s]/1 -> BasicYawStabilityControl/3(Vel_wrt_WorldSys(VehSys)[m/s])
  BasicYawStabilityControl/2(Active[0;1]) -> Switch/2
  BasicYawStabilityControl/1(WheelBrakePressures[Pa]) -> Switch/1
  WheelBrakePressuresFromBrakeHydraulics[Pa]/1 -> BasicYawStabilityControl/2(WheelBrakePressureFromBrakeHydraulics)
  Switch/1 -> Switch1/3, BasicAntiLockBrakeControl/2(RequiredWheelBrakePressures[Pa])
  BasicAntiLockBrakeControl/1(WheelBrakePressures[Pa]) -> Switch1/1
  Switch1/1 -> WheelBrakePressures[Pa]/1
  BasicAntiLockBrakeControl/2(Active[0;1]) -> Switch1/2
  BasicYawStabilityControl/3(YawStabilityControlInfo) -> YawStabilityControlInfo/1
  WheelBrakePressuresFromBrakeHydraulics[Pa]1/1 -> Switch/3
